simulink model "BLDC_w1p9"  (R2020a)
settings: Solver=VariableStepAuto  StartTime=0.0  StopTime=10.0  RelTol=1e-3
libraries: simulink x6
settings Model: Creator=avn19  LastModifiedBy=avn19

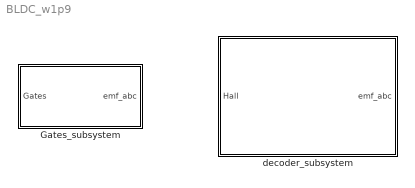
== system BLDC_w1p9 ==
  Gates_subsystem : Subsystem
  decoder_subsystem : Subsystem

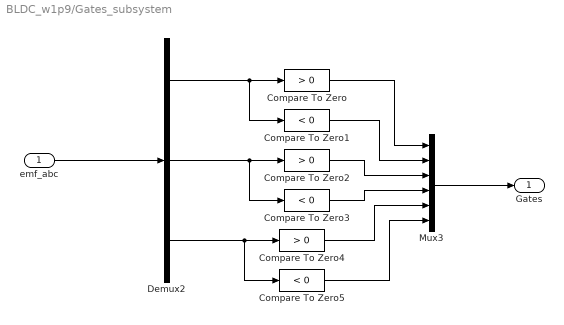
== system BLDC_w1p9/Gates_subsystem ==
  "emf_abc " : Inport
  Compare To Zero : simulink/Logic and Bit Operations/Compare To Zero  relop=>  OutDataTypeStr=boolean  ZeroCross=off
  Compare To Zero1 : simulink/Logic and Bit Operations/Compare To Zero  relop=<  OutDataTypeStr=boolean  ZeroCross=off
  Compare To Zero2 : simulink/Logic and Bit Operations/Compare To Zero  relop=>  OutDataTypeStr=boolean  ZeroCross=off
  Compare To Zero3 : simulink/Logic and Bit Operations/Compare To Zero  relop=<  OutDataTypeStr=boolean  ZeroCross=off
  Compare To Zero4 : simulink/Logic and Bit Operations/Compare To Zero  relop=>  OutDataTypeStr=boolean  ZeroCross=off
  Compare To Zero5 : simulink/Logic and Bit Operations/Compare To Zero  relop=<  OutDataTypeStr=boolean  ZeroCross=off
  Demux2 : Demux  Outputs=3
  Mux3 : Mux  Inputs=6
  Gates : Outport
  wires:
  Demux2/2 -> Compare To Zero2/1, Compare To Zero3/1
  Demux2/1 -> Compare To Zero/1, Compare To Zero1/1
  Compare To Zero1/1 -> Mux3/2
  Mux3/1 -> Gates/1
  Compare To Zero3/1 -> Mux3/4
  Compare To Zero4/1 -> Mux3/5
  Compare To Zero/1 -> Mux3/1
  "emf_abc "/1 -> Demux2/1
  Compare To Zero5/1 -> Mux3/6
  Demux2/3 -> Compare To Zero4/1, Compare To Zero5/1
  Compare To Zero2/1 -> Mux3/3

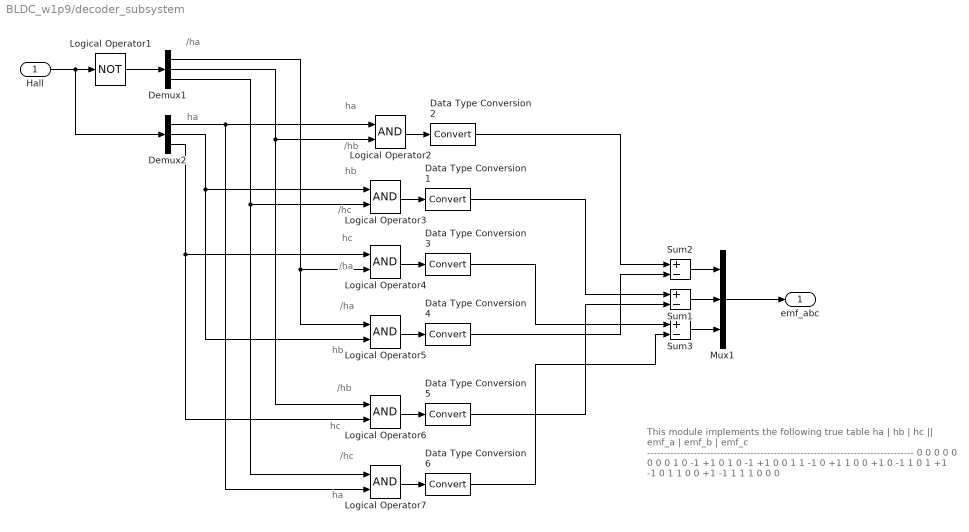
== system BLDC_w1p9/decoder_subsystem ==
  note: /hb
  note: hc
  note: ha
  note: /hc
  note: /ha
  note: ha
  note: /hc
  note: hc
  note: hb
  note: /ha
  note: hb
  note: ha
  note: /ha
  note: /hb
  note: This module implements the following true table
      |
      |    ha   |   hb   |   hc   ||   emf_a   |   emf_b   |   emf_c
      |     --------------------------------------------------------------------------------
      | 0          0         0          0               0               0
      | 0          0         1          0               -1              +1
      | 0          1         0          -1              +1                0
      | 0          1         1          -1               0               +1
      | 1          0         0         +1               0               -1
      | 1          0         1         +1              -1                0
      | 1          1         0          0              +1               -1
      | 1          1         1          0               0                0
  Hall : Inport
  Data Type Conversion{1..6} (6 alike) : DataTypeConversion
  Demux1 : Demux  Outputs=3
  Demux2 : Demux  Outputs=3
  Logical Operator1 : Logic  Operator=NOT  AllPortsSameDT=off  OutDataTypeStr=boolean
  Logical Operator{2..7} (6 alike) : Logic  AllPortsSameDT=off  OutDataTypeStr=boolean
  Mux1 : Mux  Inputs=3
  Sum1 : Sum  Inputs=+-  OutDataTypeStr=double
  Sum2 : Sum  Inputs=+-  OutDataTypeStr=double
  Sum3 : Sum  Inputs=+-  OutDataTypeStr=double
  emf_abc : Outport
  wires:
  Hall/1 -> Logical Operator1/1, Demux2/1
  Logical Operator5/1 -> Data Type Conversion4/1
  Logical Operator7/1 -> Data Type Conversion6/1
  Demux1/1 -> Logical Operator4/2, Logical Operator5/1
  Demux2/2 -> Logical Operator3/1, Logical Operator5/2
  Logical Operator6/1 -> Data Type Conversion5/1
  Logical Operator1/1 -> Demux1/1
  Demux2/3 -> Logical Operator4/1, Logical Operator6/2
  Data Type Conversion3/1 -> Sum3/1
  Demux2/1 -> Logical Operator2/1, Logical Operator7/2
  Demux1/3 -> Logical Operator3/2, Logical Operator7/1
  Logical Operator2/1 -> Data Type Conversion2/1
  Sum3/1 -> Mux1/3
  Data Type Conversion6/1 -> Sum3/2
  Data Type Conversion2/1 -> Sum2/1
  Logical Operator3/1 -> Data Type Conversion1/1
  Data Type Conversion5/1 -> Sum1/2
  Data Type Conversion4/1 -> Sum2/2
  Demux1/2 -> Logical Operator2/2, Logical Operator6/1
  Data Type Conversion1/1 -> Sum1/1
  Logical Operator4/1 -> Data Type Conversion3/1
  Sum2/1 -> Mux1/1
  Sum1/1 -> Mux1/2
  Mux1/1 -> emf_abc/1
